simulink model "car_sim"  (R2023a)
settings: Solver=FixedStepAuto  StartTime=0.0  StopTime=20  FixedStep=.01  RelTol=1e-3
values from neighbouring files (symbols this model uses):
  cg = 13/12    (= 1.08333333333)    [car_script.m]    (also in car_script_FY_lookup.m; car_script_Pacejka4.m)
  chassis_k = 1000    [car_script.m]    (also in car_script_FY_lookup.m; car_script_Pacejka4.m)
  dist = zeros(1, length(road_height_right))    [car_script_FY_lookup.m]    (also in car_script_Pacejka4.m)
  f_anti = .2    (= 0.2)    [car_script.m]    (also in car_script_FY_lookup.m; car_script_Pacejka4.m)
  f_arb = 202.9*12    (= 2434.8)    [car_script.m]    (also in car_script_FY_lookup.m; car_script_Pacejka4.m)
  f_c = f_damp_ratio*(2*sqrt(f_sprung*f_spring/(32.17*2)))    [car_script.m]    (also in car_script_FY_lookup.m; car_script_Pacejka4.m)
  f_MR_arb = .4    (= 0.4)    [car_script.m]    (also in car_script_FY_lookup.m; car_script_Pacejka4.m)
  f_MR_spring = .99    (= 0.99)    [car_script.m]    (also in car_script_FY_lookup.m; car_script_Pacejka4.m)
  f_rc = 1/12    (= 0.0833333333333)    [car_script.m]    (also in car_script_FY_lookup.m; car_script_Pacejka4.m)
  f_spring = 250*12    (= 3000)    [car_script.m]    (also in car_script_FY_lookup.m; car_script_Pacejka4.m)
  f_sprung = total_weight*weight_distribution-f_unsprung    (= 276.76)    [car_script.m]    (also in car_script_FY_lookup.m; car_script_Pacejka4.m)
  f_unsprung = 48.24    [car_script.m]    (also in car_script_FY_lookup.m; car_script_Pacejka4.m)
  f_unsprung_cg = 6/12    (= 0.5)    [car_script.m]    (also in car_script_FY_lookup.m; car_script_Pacejka4.m)
  fy_slip_angle_lookup = [fy_slip_angle_lookup, -flip(fy_slip_angle_lookup(:,1:15),2)]    [car_script.m]    (also in car_script_FY_lookup.m)
  Izz = 500    [car_script.m]    (also in car_script_FY_lookup.m; car_script_Pacejka4.m)
  r_anti = .2    (= 0.2)    [car_script.m]    (also in car_script_FY_lookup.m; car_script_Pacejka4.m)
  r_arb = 108.66*12    (= 1303.92)    [car_script.m]    (also in car_script_FY_lookup.m; car_script_Pacejka4.m)
  r_c = r_damp_ratio*(2*sqrt(r_sprung*r_spring/(32.17*2)))    [car_script.m]    (also in car_script_FY_lookup.m; car_script_Pacejka4.m)
  r_MR_arb = .25    (= 0.25)    [car_script.m]    (also in car_script_FY_lookup.m; car_script_Pacejka4.m)
  r_MR_spring = .96    (= 0.96)    [car_script.m]    (also in car_script_FY_lookup.m; car_script_Pacejka4.m)
  r_rc = 2/12    (= 0.166666666667)    [car_script.m]    (also in car_script_FY_lookup.m; car_script_Pacejka4.m)
  r_spring = 150*12    (= 1800)    [car_script.m]    (also in car_script_FY_lookup.m; car_script_Pacejka4.m)
  r_sprung = total_weight*weight_distribution-r_unsprung    (= 277.44)    [car_script.m]    (also in car_script_FY_lookup.m; car_script_Pacejka4.m)
  r_unsprung = 47.56    [car_script.m]    (also in car_script_FY_lookup.m; car_script_Pacejka4.m)
  r_unsprung_cg = 6/12    (= 0.5)    [car_script.m]    (also in car_script_FY_lookup.m; car_script_Pacejka4.m)
  road_height_left = [zeros(1,10000)]    [car_script.m]    (also in car_script_FY_lookup.m; car_script_Pacejka4.m)
  road_height_right = [zeros(1,10000)]    [car_script.m]    (also in car_script_FY_lookup.m; car_script_Pacejka4.m)
  timestep = .01    (= 0.01)    [car_script.m]    (also in car_script_FY_lookup.m; car_script_Pacejka4.m)
  tire_c = .1*(2*sqrt(tire_k*f_unsprung/(2*32.17)))    [car_script.m]    (also in car_script_FY_lookup.m; car_script_Pacejka4.m)
  tire_k = 989*12    (= 11868)    [car_script.m]    (also in car_script_FY_lookup.m; car_script_Pacejka4.m)
  total_unsprung = f_unsprung + r_unsprung    (= 95.8)    [car_script.m]    (also in car_script_FY_lookup.m; car_script_Pacejka4.m)
  total_weight = 650    [car_script.m]    (also in car_script_FY_lookup.m; car_script_Pacejka4.m)
  track = 48/12    (= 4)    [car_script.m]    (also in car_script_FY_lookup.m; car_script_Pacejka4.m)
  vx_o = 51.3333    [car_script.m]    (also in car_script_FY_lookup.m; car_script_Pacejka4.m = 51.33)
  wheelbase = 60.5/12    (= 5.04166666667)    [car_script.m]    (also in car_script_FY_lookup.m; car_script_Pacejka4.m)
libraries: simulink_extras x1, simulink x1
(part 1 of 2)
settings Model: PauseTimes=1.01  Creator=truma  LastModifiedBy=truma
settings SolverCC: ZeroCrossAlgorithm=Adaptive
settings DebuggingCC: MaskedZcDiagnostic=none  IgnoredZcDiagnostic=none  ParameterPrecisionLossMsg=none  UnderSpecifiedDimensionMsg=warning

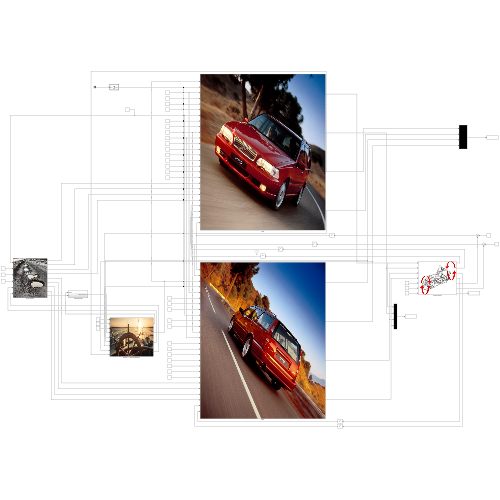
[thumbnail: Simulink's stored preview of the top-level diagram]
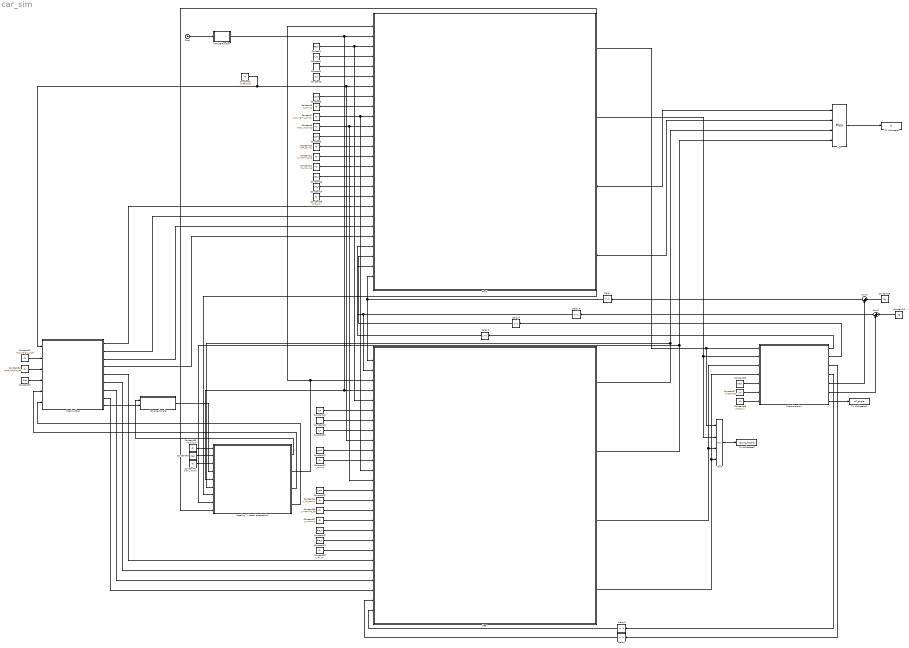
== system car_sim ==
  Chassis torsion : Subsystem
      mask Display: image('torsion.jpg'); % Use "Edit Image" on toolstrip to change.
  Clock : Clock
  Constant : Constant  Value=track
  Constant1 : Constant  Value=f_rc
  Constant10 : Constant  Value=f_MR_spring
  Constant11 : Constant  Value=f_unsprung_cg
  Constant12 : Constant  Value=f_unsprung
  Constant13 : Constant  Value=tire_k
  Constant14 : Constant  Value=tire_c
  Constant15 : Constant  Value=cg
  Constant16 : Constant  Value=f_MR_arb
  Constant18 : Constant  Value=r_rc
  Constant19 : Constant  Value=r_spring
  Constant2 : Constant  Value=f_spring
  Constant20 : Constant  Value=r_c
  Constant21 : Constant  Value=r_anti
  Constant22 : Constant  Value=r_sprung
  Constant23 : Constant  Value=cg
  Constant24 : Constant  Value=r_MR_spring
  Constant25 : Constant  Value=r_arb
  Constant26 : Constant  Value=r_unsprung_cg
  Constant27 : Constant  Value=r_unsprung
  Constant28 : Constant  Value=tire_k
  Constant29 : Constant  Value=tire_c
  Constant3 : Constant  Value=f_c
  Constant30 : Constant  Value=r_MR_arb
  Constant31 : Constant  Value=road_height_right
  Constant32 : Constant  Value=road_height_left
  Constant33 : Constant  Value=dist
  Constant36 : Constant  Value=track
  Constant37 : Constant  Value=wheelbase
  Constant38 : Constant  Value=chassis_k
  Constant39 : Constant  Value=wheelbase
  Constant4 : Constant  Value=wheelbase
  Constant40 : Constant  Value=track
  Constant41 : Constant  Value=total_weight
  Constant5 : Constant  Value=f_anti
  Constant6 : Constant  Value=f_sprung
  Constant7 : Constant  Value=f_sprung+r_sprung
  Constant8 : Constant  Value=total_unsprung
  Constant9 : Constant  Value=f_arb
  Delay : Delay  DelayLength=1  InitialCondition=cg
  Delay{2..5} (4 alike) : Delay  DelayLength=1
  Delay8 : Delay  DelayLength=1  InitialCondition=cg
  Front : Subsystem
      mask Display: image('front.jpg'); % Use "Edit Image" on toolstrip to change.
  MATLAB Function : MATLAB Function  TreatAsAtomicUnit=on
  Mux : Mux
  Mux1 : Mux
  Rear : Subsystem
      mask Display: image('rear.jpg'); % Use "Edit Image" on toolstrip to change.
  Road surface : Subsystem
      mask Display: image('pothole.jpg'); % Use "Edit Image" on toolstrip to change.
  Sum2 : Sum  Inputs=|++
  Sum3 : Sum  Inputs=|++
  To Workspace : ToWorkspace  VariableName=Fz  SaveFormat=Timeseries  SampleTime=-1
  To Workspace1 : ToWorkspace  VariableName=roll_angle  SaveFormat=Timeseries  SampleTime=-1
  To Workspace2 : ToWorkspace  VariableName=sprung_heights  SaveFormat=Timeseries  SampleTime=-1
  "steering -> lateral acceleration" : Subsystem
      mask Display: image('steering.jpeg'); % Use "Edit Image" on toolstrip to change.
  traversed angle : Subsystem
  wires:
  Front/2(sprung height FL) -> Mux1/2, Chassis torsion/2(sprung height FL)
  Rear/4(sprung height RL) -> Chassis torsion/4(sprung height RL), Mux1/4
  Chassis torsion/1(FR) -> Delay5/1
  Chassis torsion/2(FL) -> Delay4/1
  Chassis torsion/3(RR) -> Delay2/1
  Chassis torsion/4(RL) -> Delay3/1
  Constant/1 -> Rear/5(track), Front/3(track)
  Constant2/1 -> Front/5(front spring stiff)
  Constant3/1 -> Front/6(front damping coefficient)
  Constant5/1 -> Front/8(anti-squat)
  Constant6/1 -> Front/9(front sprung weight)
  Constant7/1 -> Front/10(total sprung weight), Rear/12(total sprung weight)
  Constant8/1 -> Front/11(total unsprung weight), Rear/13(total unsprung weight)
  Constant9/1 -> Front/12(front roll bar stiffness)
  Constant10/1 -> Front/13(front spring MR)
  Constant11/1 -> Front/14(front unsprung cg)
  Constant12/1 -> Front/15(front unsprung weight)
  Constant13/1 -> Front/16(front tire stiffness)
  Constant14/1 -> Front/17(front tire damping)
  Constant16/1 -> Front/18(front arb MR)
  Constant18/1 -> Rear/6(rear RC)
  Constant19/1 -> Rear/7(rear spring stiff)
  Constant20/1 -> Rear/8(rear damping coefficient)
  Constant21/1 -> Rear/10(anti-dive)
  Constant22/1 -> Rear/11(rear sprung weight)
  Constant25/1 -> Rear/14(rear roll bar stiffness)
  Constant24/1 -> Rear/15(rear spring MR)
  Constant26/1 -> Rear/16(rear unsprung cg)
  Constant27/1 -> Rear/17(rear unsprung weight)
  Constant28/1 -> Rear/18(rear tire stiffness)
  Constant29/1 -> Rear/19(rear tire damping)
  Constant30/1 -> Rear/20(rear arb MR)
  Road surface/1(FR_surface) -> Front/19(road height FR)
  Road surface/3(FL_surface) -> Front/21(road height FL)
  Road surface/7(RL_surface) -> Rear/23(road height RL)
  Road surface/5(RR_surface) -> Rear/21(road height RR)
  Road surface/2(FR_vel) -> Front/20(road velocity FR)
  Road surface/6(RR_vel) -> Rear/22(road velocity RR)
  Road surface/4(FL_vel) -> Front/22(road velocity FL)
  Road surface/8(RL_vel) -> Rear/24(road velocity RL)
  Constant31/1 -> Road surface/2(road height right)
  Constant32/1 -> Road surface/3(road height left)
  Constant33/1 -> Road surface/4(dist)
  Constant4/1 -> Road surface/1(wheelbase), Rear/9(wheelbase), Front/7(wheelbase)
  Front/4(Fz_FL) -> Mux/2, "steering -> lateral acceleration"/7(Fz_fl)
  Rear/1(Fz_RR) -> Mux/3, "steering -> lateral acceleration"/6(Fz_rr)
  Rear/2(Fz_RL) -> "steering -> lateral acceleration"/8(Fz_rl), Mux/4
  Mux/1 -> To Workspace/1
  Constant36/1 -> Chassis torsion/5(track)
  Constant38/1 -> Chassis torsion/7(chassis torsional stiffness)
  Constant37/1 -> Chassis torsion/6(wheelbase)
  Delay3/1 -> Rear/26(RL chassis force)
  Delay2/1 -> Rear/25(RR chassis force)
  Delay5/1 -> Front/23(FR chassis force)
  Delay4/1 -> Front/24(FL chassis force)
  Constant39/1 -> "steering -> lateral acceleration"/1(wheelbase)
  Constant40/1 -> "steering -> lateral acceleration"/2(track)
  Constant41/1 -> "steering -> lateral acceleration"/3(total_weight)
  Chassis torsion/7(roll) -> To Workspace1/1
  Clock/1 -> MATLAB Function/1(time)
  MATLAB Function/1(long_a) -> "steering -> lateral acceleration"/5(long_a), Rear/4(longitudinal a), Front/2(longitudinal a)
  Delay/1 -> Front/26(CG h), Rear/1(CG_front)
  Constant23/1 -> Sum2/1
  Sum2/1 -> Delay/1
  "steering -> lateral acceleration"/2(lat_a) -> Front/1(lateral a), Rear/3(lateral a)
  Chassis torsion/5(CG_f) -> Sum2/2
  Front/1(sprung height FR) -> Mux1/1, Chassis torsion/1(sprung height FR)
  Rear/3(sprung height RR) -> Mux1/3, Chassis torsion/3(sprung height RR)
  Mux1/1 -> To Workspace2/1
  Constant1/1 -> Front/4(front RC)
  Sum3/1 -> Delay8/1
  Constant15/1 -> Sum3/1
  Chassis torsion/6(CG_r) -> Sum3/2
  Delay8/1 -> Front/25(CG_rear), Rear/2(CG h)
  "steering -> lateral acceleration"/1(radius) -> traversed angle/1(radius)
  traversed angle/1(theta_world_frame) -> "steering -> lateral acceleration"/4(theta)
  Road surface/9(v) -> traversed angle/2(v)
  "steering -> lateral acceleration"/4(y_v) -> Road surface/6(y_v)
  "steering -> lateral acceleration"/3(x_v) -> Road surface/5(x_v)
  Front/3(Fz_FR) -> Mux/1, "steering -> lateral acceleration"/9(Fz_fr)

== system car_sim/Chassis torsion ==
  sprung height FR : Inport
  sprung height FL : Inport  Port=2
  sprung height RR : Inport  Port=3
  sprung height RL : Inport  Port=4
  track : Inport  Port=5
  wheelbase : Inport  Port=6
  chassis torsional stiffness : Inport  Port=7
  MATLAB Function : MATLAB Function  TreatAsAtomicUnit=on
  FR : Outport
  FL : Outport  Port=2
  RR : Outport  Port=3
  RL : Outport  Port=4
  CG_f : Outport  Port=5
  CG_r : Outport  Port=6
  roll : Outport  Port=7
  wires:
  sprung height FR/1 -> MATLAB Function/1(sprung_height_FR)
  sprung height FL/1 -> MATLAB Function/2(sprung_height_FL)
  sprung height RR/1 -> MATLAB Function/3(sprung_height_RR)
  sprung height RL/1 -> MATLAB Function/4(sprung_height_RL)
  track/1 -> MATLAB Function/5(track)
  wheelbase/1 -> MATLAB Function/7(wheelbase)
  chassis torsional stiffness/1 -> MATLAB Function/6(chassis_torsional_stiffness)
  MATLAB Function/2(FL) -> FL/1
  MATLAB Function/3(RR) -> RR/1
  MATLAB Function/4(RL) -> RL/1
  MATLAB Function/5(CG_f) -> CG_f/1
  MATLAB Function/7(roll) -> roll/1
  MATLAB Function/6(CG_r) -> CG_r/1
  MATLAB Function/1(FR) -> FR/1

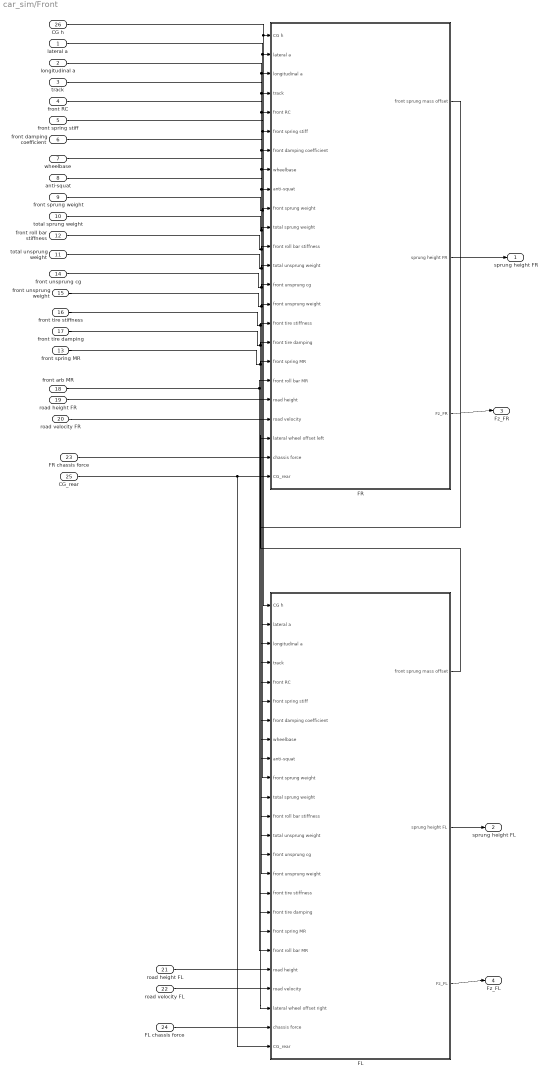
== system car_sim/Front ==
  lateral a : Inport
  longitudinal a : Inport  Port=2
  track : Inport  Port=3
  front RC : Inport  Port=4
  front spring stiff : Inport  Port=5
  front damping coefficient : Inport  Port=6
  wheelbase : Inport  Port=7
  anti-squat : Inport  Port=8
  front sprung weight : Inport  Port=9
  total sprung weight : Inport  Port=10
  total unsprung weight : Inport  Port=11
  front roll bar stiffness : Inport  Port=12
  front spring MR : Inport  Port=13
  front unsprung cg : Inport  Port=14
  front unsprung weight : Inport  Port=15
  front tire stiffness : Inport  Port=16
  front tire damping : Inport  Port=17
  front arb MR : Inport  Port=18
  road height FR : Inport  Port=19
  road velocity FR : Inport  Port=20
  road height FL : Inport  Port=21
  road velocity FL : Inport  Port=22
  FR chassis force : Inport  Port=23
  FL chassis force : Inport  Port=24
  CG_rear : Inport  Port=25
  CG h : Inport  Port=26
  FL : Subsystem
  FR : Subsystem
  sprung height FR : Outport
  sprung height FL : Outport  Port=2
  Fz_FR : Outport  Port=3
  Fz_FL : Outport  Port=4
  wires:
  CG h/1 -> FL/1(CG h), FR/1(CG h)
  lateral a/1 -> FL/2(lateral a), FR/2(lateral a)
  longitudinal a/1 -> FL/3(longitudinal a), FR/3(longitudinal a)
  track/1 -> FL/4(track), FR/4(track)
  front RC/1 -> FL/5(front RC), FR/5(front RC)
  front spring stiff/1 -> FL/6(front spring stiff), FR/6(front spring stiff)
  front damping coefficient/1 -> FL/7(front damping coefficient), FR/7(front damping coefficient)
  wheelbase/1 -> FL/8(wheelbase), FR/8(wheelbase)
  anti-squat/1 -> FL/9(anti-squat), FR/9(anti-squat)
  front sprung weight/1 -> FL/10(front sprung weight), FR/10(front sprung weight)
  total sprung weight/1 -> FL/11(total sprung weight), FR/11(total sprung weight)
  total unsprung weight/1 -> FL/13(total unsprung weight), FR/13(total unsprung weight)
  front roll bar stiffness/1 -> FL/12(front roll bar stiffness), FR/12(front roll bar stiffness)
  FR/1(front sprung mass offset) -> FL/22(lateral wheel offset right)
  front spring MR/1 -> FL/18(front spring MR), FR/18(front spring MR)
  front unsprung cg/1 -> FL/14(front unsprung cg), FR/14(front unsprung cg)
  front unsprung weight/1 -> FL/15(front unsprung weight), FR/15(front unsprung weight)
  front tire stiffness/1 -> FL/16(front tire stiffness), FR/16(front tire stiffness)
  front tire damping/1 -> FL/17(front tire damping), FR/17(front tire damping)
  front arb MR/1 -> FL/19(front roll bar MR), FR/19(front roll bar MR)
  FL/1(front sprung mass offset) -> FR/22(lateral wheel offset left)
  road height FR/1 -> FR/20(road height)
  road velocity FR/1 -> FR/21(road velocity)
  road height FL/1 -> FL/20(road height)
  road velocity FL/1 -> FL/21(road velocity)
  FR/2(sprung height FR) -> sprung height FR/1
  FL/2(sprung height FL) -> sprung height FL/1
  FR chassis force/1 -> FR/23(chassis force)
  FL chassis force/1 -> FL/23(chassis force)
  FR/3(Fz_FR) -> Fz_FR/1
  FL/3(Fz_FL) -> Fz_FL/1
  CG_rear/1 -> FL/24(CG_rear), FR/24(CG_rear)

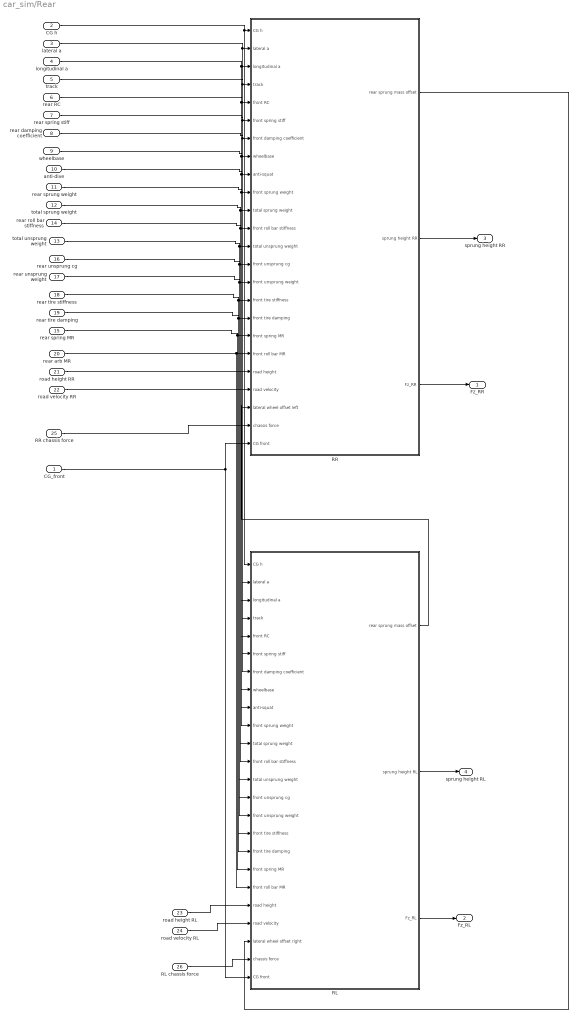
== system car_sim/Rear ==
  CG_front : Inport
  CG h : Inport  Port=2
  lateral a : Inport  Port=3
  longitudinal a : Inport  Port=4
  track : Inport  Port=5
  rear RC : Inport  Port=6
  rear spring stiff : Inport  Port=7
  rear damping coefficient : Inport  Port=8
  wheelbase : Inport  Port=9
  anti-dive : Inport  Port=10
  rear sprung weight : Inport  Port=11
  total sprung weight : Inport  Port=12
  total unsprung weight : Inport  Port=13
  rear roll bar stiffness : Inport  Port=14
  rear spring MR : Inport  Port=15
  rear unsprung cg : Inport  Port=16
  rear unsprung weight : Inport  Port=17
  rear tire stiffness : Inport  Port=18
  rear tire damping : Inport  Port=19
  rear arb MR : Inport  Port=20
  road height RR : Inport  Port=21
  road velocity RR : Inport  Port=22
  road height RL : Inport  Port=23
  road velocity RL : Inport  Port=24
  RR chassis force : Inport  Port=25
  RL chassis force : Inport  Port=26
  RL : Subsystem
  RR : Subsystem
  Fz_RR : Outport
  Fz_RL : Outport  Port=2
  sprung height RR : Outport  Port=3
  sprung height RL : Outport  Port=4
  wires:
  CG h/1 -> RL/1(CG h), RR/1(CG h)
  lateral a/1 -> RL/2(lateral a), RR/2(lateral a)
  longitudinal a/1 -> RL/3(longitudinal a), RR/3(longitudinal a)
  track/1 -> RL/4(track), RR/4(track)
  rear RC/1 -> RL/5(front RC), RR/5(front RC)
  rear spring stiff/1 -> RL/6(front spring stiff), RR/6(front spring stiff)
  rear damping coefficient/1 -> RL/7(front damping coefficient), RR/7(front damping coefficient)
  wheelbase/1 -> RL/8(wheelbase), RR/8(wheelbase)
  anti-dive/1 -> RL/9(anti-squat), RR/9(anti-squat)
  rear sprung weight/1 -> RL/10(front sprung weight), RR/10(front sprung weight)
  total sprung weight/1 -> RL/11(total sprung weight), RR/11(total sprung weight)
  total unsprung weight/1 -> RL/13(total unsprung weight), RR/13(total unsprung weight)
  rear roll bar stiffness/1 -> RL/12(front roll bar stiffness), RR/12(front roll bar stiffness)
  RR/1(rear sprung mass offset) -> RL/22(lateral wheel offset right)
  rear spring MR/1 -> RL/18(front spring MR), RR/18(front spring MR)
  rear unsprung cg/1 -> RL/14(front unsprung cg), RR/14(front unsprung cg)
  rear unsprung weight/1 -> RL/15(front unsprung weight), RR/15(front unsprung weight)
  rear tire stiffness/1 -> RL/16(front tire stiffness), RR/16(front tire stiffness)
  rear tire damping/1 -> RL/17(front tire damping), RR/17(front tire damping)
  rear arb MR/1 -> RL/19(front roll bar MR), RR/19(front roll bar MR)
  RL/1(rear sprung mass offset) -> RR/22(lateral wheel offset left)
  road height RR/1 -> RR/20(road height)
  road velocity RR/1 -> RR/21(road velocity)
  road height RL/1 -> RL/20(road height)
  road velocity RL/1 -> RL/21(road velocity)
  RR/2(sprung height RR) -> sprung height RR/1
  RL/2(sprung height RL) -> sprung height RL/1
  RR chassis force/1 -> RR/23(chassis force)
  RL chassis force/1 -> RL/23(chassis force)
  RR/3(Fz_RR) -> Fz_RR/1
  RL/3(Fz_RL) -> Fz_RL/1
  CG_front/1 -> RL/24(CG front), RR/24(CG front)

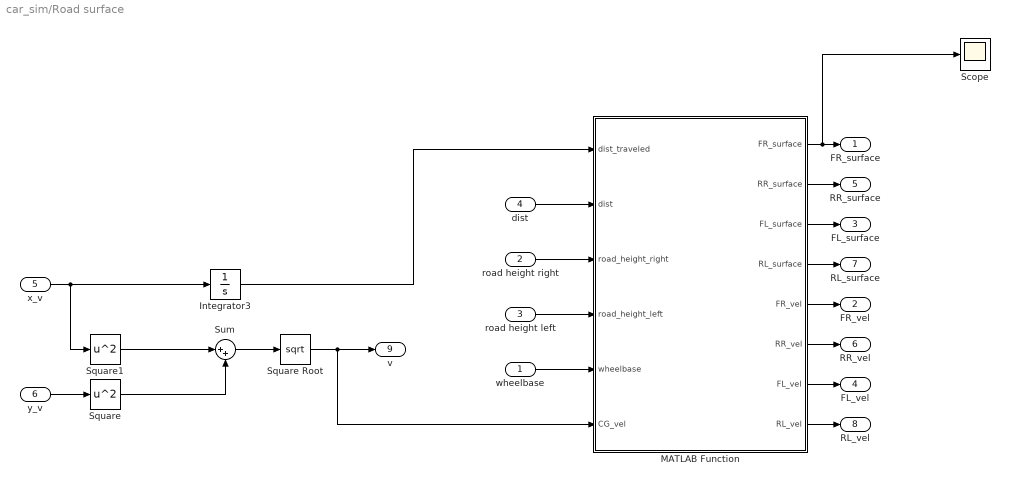
== system car_sim/Road surface ==
  wheelbase : Inport
  road height right : Inport  Port=2
  road height left : Inport  Port=3
  dist : Inport  Port=4
  x_v : Inport  Port=5
  y_v : Inport  Port=6
  Integrator3 : Integrator
  MATLAB Function : MATLAB Function  TreatAsAtomicUnit=on
  Scope : Scope
  Square : Math  Operator=square
  Square Root : Sqrt
  Square1 : Math  Operator=square
  Sum : Sum  Inputs=|++
  FR_surface : Outport
  FR_vel : Outport  Port=2
  FL_surface : Outport  Port=3
  FL_vel : Outport  Port=4
  RR_surface : Outport  Port=5
  RR_vel : Outport  Port=6
  RL_surface : Outport  Port=7
  RL_vel : Outport  Port=8
  v : Outport  Port=9
  wires:
  Integrator3/1 -> MATLAB Function/1(dist_traveled)
  road height right/1 -> MATLAB Function/3(road_height_right)
  road height left/1 -> MATLAB Function/4(road_height_left)
  dist/1 -> MATLAB Function/2(dist)
  wheelbase/1 -> MATLAB Function/5(wheelbase)
  MATLAB Function/1(FR_surface) -> FR_surface/1, Scope/1
  MATLAB Function/2(RR_surface) -> RR_surface/1
  MATLAB Function/3(FL_surface) -> FL_surface/1
  MATLAB Function/4(RL_surface) -> RL_surface/1
  x_v/1 -> Integrator3/1, Square1/1
  MATLAB Function/8(RL_vel) -> RL_vel/1
  MATLAB Function/7(FL_vel) -> FL_vel/1
  MATLAB Function/6(RR_vel) -> RR_vel/1
  MATLAB Function/5(FR_vel) -> FR_vel/1
  y_v/1 -> Square/1
  Square1/1 -> Sum/1
  Square/1 -> Sum/2
  Sum/1 -> Square Root/1
  Square Root/1 -> MATLAB Function/6(CG_vel), v/1

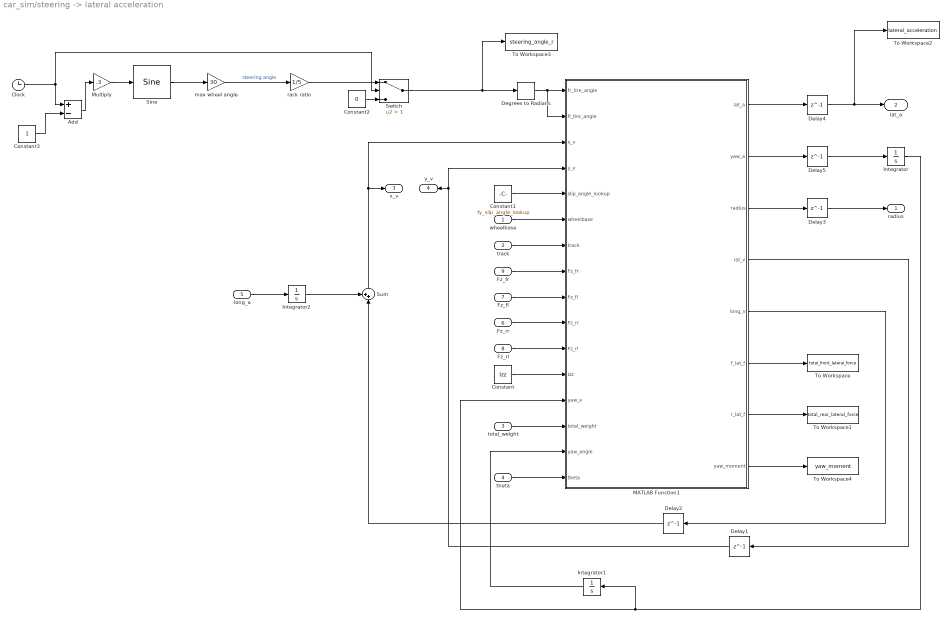
== system car_sim/steering -> lateral acceleration ==
  wheelbase : Inport
  track : Inport  Port=2
  total_weight : Inport  Port=3
  theta : Inport  Port=4
  long_a : Inport  Port=5
  Fz_rr : Inport  Port=6
  Fz_fl : Inport  Port=7
  Fz_rl : Inport  Port=8
  Fz_fr : Inport  Port=9
  Add : Sum  Inputs=+-
  Clock : Clock
  Constant : Constant  Value=Izz
  Constant1 : Constant  Value=fy_slip_angle_lookup
  Constant2 : Constant  Value=0
  Constant3 : Constant
  Degrees to Radians : simulink_extras/Transformations/Degrees to Radians
  Delay{1,3..5} (4 alike) : Delay  DelayLength=1
  Delay2 : Delay  DelayLength=1  InitialCondition=vx_o/2
  Integrator : Integrator
  Integrator1 : Integrator
  Integrator2 : Integrator
  MATLAB Function1 : MATLAB Function  TreatAsAtomicUnit=on
  Multiply : Gain  Gain=.3
  Sine : simulink/Lookup Tables/Sine  Formula=sin(2*pi*u)  NumDataPoints=(2^5)+1  OutputWordLength=16  InternalRulePriority=Speed
  Sum : Sum  Inputs=++|
  Switch : Switch  Criteria=u2 > Threshold  Threshold=1  SaturateOnIntegerOverflow=off  InputSameDT=off
  To Workspace : ToWorkspace  VariableName=total_front_lateral_force  SaveFormat=Timeseries  SampleTime=-1
  To Workspace1 : ToWorkspace  VariableName=total_rear_lateral_force  SaveFormat=Timeseries  SampleTime=-1
  To Workspace2 : ToWorkspace  VariableName=lateral_acceleration  SaveFormat=Timeseries  SampleTime=-1
  To Workspace3 : ToWorkspace  VariableName=steering_angle_r  SaveFormat=Timeseries  SampleTime=-1
  To Workspace4 : ToWorkspace  VariableName=yaw_moment  SaveFormat=Timeseries  SampleTime=-1
  max wheel angle : Gain  Gain=30
  rack ratio : Gain  Gain=1/5
  radius : Outport
  lat_a : Outport  Port=2
  x_v : Outport  Port=3
  y_v : Outport  Port=4
  wires:
  Multiply/1 -> Sine/1
  max wheel angle/1 -> rack ratio/1  "steering angle"
  Sine/1 -> max wheel angle/1
  Clock/1 -> Add/1, Switch/2
  Constant/1 -> MATLAB Function1/12(Izz)
  Constant1/1 -> MATLAB Function1/5(slip_angle_lookup)
  Fz_fr/1 -> MATLAB Function1/8(Fz_fr)
  wheelbase/1 -> MATLAB Function1/6(wheelbase)
  Fz_fl/1 -> MATLAB Function1/9(Fz_fl)
  MATLAB Function1/2(yaw_a) -> Delay5/1
  Integrator/1 -> MATLAB Function1/13(yaw_v), Integrator1/1
  total_weight/1 -> MATLAB Function1/14(total_weight)
  track/1 -> MATLAB Function1/7(track)
  rack ratio/1 -> Switch/1
  Constant2/1 -> Switch/3
  Constant3/1 -> Add/2
  Add/1 -> Multiply/1
  Switch/1 -> To Workspace3/1, Degrees to Radians/1
  MATLAB Function1/3(radius) -> Delay3/1
  MATLAB Function1/4(lat_v) -> Delay1/1
  Delay1/1 -> MATLAB Function1/4(y_v), y_v/1
  MATLAB Function1/5(long_v) -> Delay2/1
  long_a/1 -> Integrator2/1
  Delay2/1 -> Sum/2
  Integrator2/1 -> Sum/1
  Sum/1 -> x_v/1, MATLAB Function1/3(x_v)
  Delay3/1 -> radius/1
  Delay4/1 -> To Workspace2/1, lat_a/1
  MATLAB Function1/1(lat_a) -> Delay4/1
  Delay5/1 -> Integrator/1
  theta/1 -> MATLAB Function1/16(theta)
  MATLAB Function1/6(f_lat_f) -> To Workspace/1
  MATLAB Function1/7(r_lat_f) -> To Workspace1/1
  Fz_rr/1 -> MATLAB Function1/10(Fz_rr)
  Fz_rl/1 -> MATLAB Function1/11(Fz_rl)
  Integrator1/1 -> MATLAB Function1/15(yaw_angle)
  Degrees to Radians/1 -> MATLAB Function1/2(fl_tire_angle), MATLAB Function1/1(fr_tire_angle)
  MATLAB Function1/8(yaw_moment) -> To Workspace4/1

== system car_sim/traversed angle ==
  radius : Inport
  v : Inport  Port=2
  Delay : Delay  DelayLength=1
  Divide : Product  Inputs=*/
  Gain : Gain  Gain=timestep
  MATLAB Function : MATLAB Function  TreatAsAtomicUnit=on
  Sum : Sum  Inputs=|++
  theta_world_frame : Outport
  wires:
  v/1 -> Gain/1
  Gain/1 -> Divide/1
  Delay/1 -> Sum/2
  Divide/1 -> Sum/1
  MATLAB Function/1(y) -> Divide/2
  Sum/1 -> Delay/1, theta_world_frame/1
  radius/1 -> MATLAB Function/1(u)

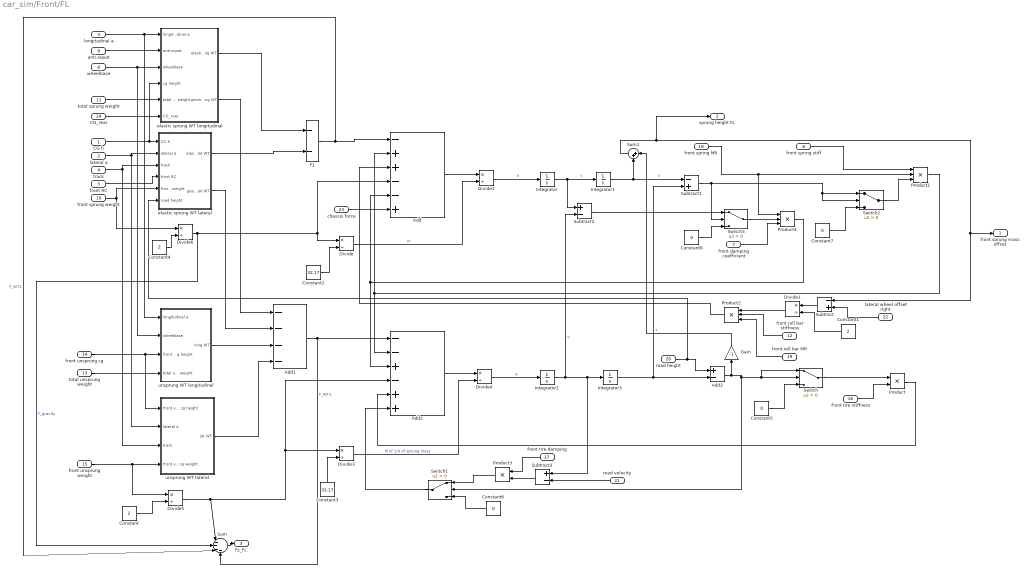
== system car_sim/Front/FL ==
  CG h : Inport
  lateral a : Inport  Port=2
  longitudinal a : Inport  Port=3
  track : Inport  Port=4
  front RC : Inport  Port=5
  front spring stiff : Inport  Port=6
  front damping coefficient : Inport  Port=7
  wheelbase : Inport  Port=8
  anti-squat : Inport  Port=9
  front sprung weight : Inport  Port=10
  total sprung weight : Inport  Port=11
  front roll bar stiffness : Inport  Port=12
  total unsprung weight : Inport  Port=13
  front unsprung cg : Inport  Port=14
  front unsprung weight : Inport  Port=15
  front tire stiffness : Inport  Port=16
  front tire damping : Inport  Port=17
  front spring MR : Inport  Port=18
  front roll bar MR : Inport  Port=19
  road height : Inport  Port=20
  road velocity : Inport  Port=21
  lateral wheel offset right : Inport  Port=22
  chassis force : Inport  Port=23
  CG_rear : Inport  Port=24
  " unsprung WT longitudinal" : Subsystem
  Add : Sum  Inputs=-++--+
  Add1 : Sum  Inputs=----
  Add2 : Sum  Inputs=--+-++
  Add3 : Sum  Inputs=+-
  Constant : Constant  Value=2
  Constant1 : Constant  Value=2
  Constant2 : Constant  Value=32.17
  Constant3 : Constant  Value=32.17
  Constant4 : Constant  Value=2
  Constant{5..8} (4 alike) : Constant  Value=0
  Divide{,1..6} (7 alike) : Product  Inputs=*/
  F1 : Sum  Inputs=--
  Gain : Gain  Gain=-1
  Integrator{,1..3} (4 alike) : Integrator
  Product : Product
  Product1 : Product  Inputs=3
  Product2 : Product  Inputs=3
  Product3 : Product
  Product4 : Product  Inputs=3
  Subtract : Sum  Inputs=-+
  Subtract1 : Sum  Inputs=-+
  Subtract2 : Sum  Inputs=+-
  Subtract3 : Sum  Inputs=+-
  Sum : Sum  Inputs=|----
  Sum1 : Sum  Inputs=|++
  Switch{,1..3} (4 alike) : Switch  Criteria=u2 > Threshold  SaturateOnIntegerOverflow=off  InputSameDT=off
  elastic sprung WT lateral : Subsystem
  elastic sprung WT longitudinal : Subsystem
  unsprung WT lateral : Subsystem
  front sprung mass offset : Outport
  sprung height FL : Outport  Port=2
  Fz_FL : Outport  Port=3
  wires:
  CG h/1 -> elastic sprung WT longitudinal/4(cg height), elastic sprung WT lateral/1(CG h)
  F1/1 -> Sum/3, Add/1  "F_WT2"
  lateral a/1 -> unsprung WT lateral/2(lateral a), elastic sprung WT lateral/2(lateral a)
  elastic sprung WT longitudinal/1(elastic long WT) -> F1/1
  wheelbase/1 -> " unsprung WT longitudinal"/2(wheelbase), elastic sprung WT longitudinal/3(wheelbase)
  anti-squat/1 -> elastic sprung WT longitudinal/2(anti-squat)
  longitudinal a/1 -> " unsprung WT longitudinal"/1(longitudinal a), elastic sprung WT longitudinal/1(longitudinal a)
  front damping coefficient/1 -> Product4/3
  lateral wheel offset right/1 -> Subtract/2
  front RC/1 -> elastic sprung WT lateral/4(front RC)
  track/1 -> unsprung WT lateral/3(track), elastic sprung WT lateral/3(track)
  front roll bar stiffness/1 -> Product2/2
  elastic sprung WT lateral/1(elastic lat WT) -> F1/2
  front spring stiff/1 -> Product1/1
  Subtract/1 -> Divide1/1
  Constant1/1 -> Divide1/2
  Divide1/1 -> Product2/1
  front sprung weight/1 -> Divide6/1, elastic sprung WT lateral/5(front sprung weight)
  Constant2/1 -> Divide/2
  Divide/1 -> Divide2/2  "m"
  Add/1 -> Divide2/1
  Divide2/1 -> Integrator/1  "a"
  Integrator/1 -> Subtract2/1, Integrator1/1  "v"
  Integrator1/1 -> Subtract1/1, Sum1/2  "x"
  total unsprung weight/1 -> " unsprung WT longitudinal"/4(total unsprung weight)
  front unsprung cg/1 -> unsprung WT lateral/1(front unsprung cg height), " unsprung WT longitudinal"/3(front unsprung weight cg height)
  elastic sprung WT longitudinal/2(geom long WT) -> Add1/1
  elastic sprung WT lateral/2(geom lat WT) -> Add1/2
  " unsprung WT longitudinal"/1(long WT) -> Add1/3
  unsprung WT lateral/1(lat WT) -> Add1/4
  Add1/1 -> Sum/4, Add2/1  "F_WT1"
  Constant3/1 -> Divide3/2
  Divide3/1 -> Divide4/2  "M of 1/4 of sprung mass"
  Add2/1 -> Divide4/1
  front unsprung weight/1 -> Divide5/1, unsprung WT lateral/4(front unsprung weight)
  Constant/1 -> Divide5/2
  Divide5/1 -> Add2/4, Divide3/1, Sum/1
  Constant4/1 -> Divide6/2
  Divide6/1 -> Sum/2, Add/4, Divide/1  "F_gravity"
  Divide4/1 -> Integrator2/1  "a"
  Integrator2/1 -> Subtract2/2, Subtract3/1, Integrator3/1  "v"
  Integrator3/1 -> Subtract1/2, Add3/2  "x"
  front spring MR/1 -> Product4/1, Product1/2
  front roll bar MR/1 -> Product2/3
  Product2/1 -> Add/3
  Product4/1 -> Add2/3, Add/5
  Product1/1 -> Add2/2, Add/2
  road height/1 -> elastic sprung WT lateral/6(road height), Add3/1
  front tire stiffness/1 -> Product/2
  Product/1 -> Add2/5
  road velocity/1 -> Subtract3/2
  Subtract3/1 -> Product3/2
  front tire damping/1 -> Product3/1
  Constant5/1 -> Switch/3
  Switch/1 -> Product/1
  Constant6/1 -> Switch1/3
  Add3/1 -> Switch1/2, Switch/1, Switch/2, Gain/1
  Product3/1 -> Switch1/1
  Switch1/1 -> Add2/6
  Subtract1/1 -> Switch2/2, Switch2/1, Switch3/2
  Constant7/1 -> Switch2/3
  Switch2/1 -> Product1/3
  Constant8/1 -> Switch3/3
  Subtract2/1 -> Switch3/1
  Switch3/1 -> Product4/2
  Sum/1 -> Fz_FL/1
  Sum1/1 -> front sprung mass offset/1, Subtract/1, sprung height FL/1
  chassis force/1 -> Add/6
  CG_rear/1 -> elastic sprung WT longitudinal/6(CG_rear)
  total sprung weight/1 -> elastic sprung WT longitudinal/5(total sprung weight)
  Gain/1 -> Sum1/1

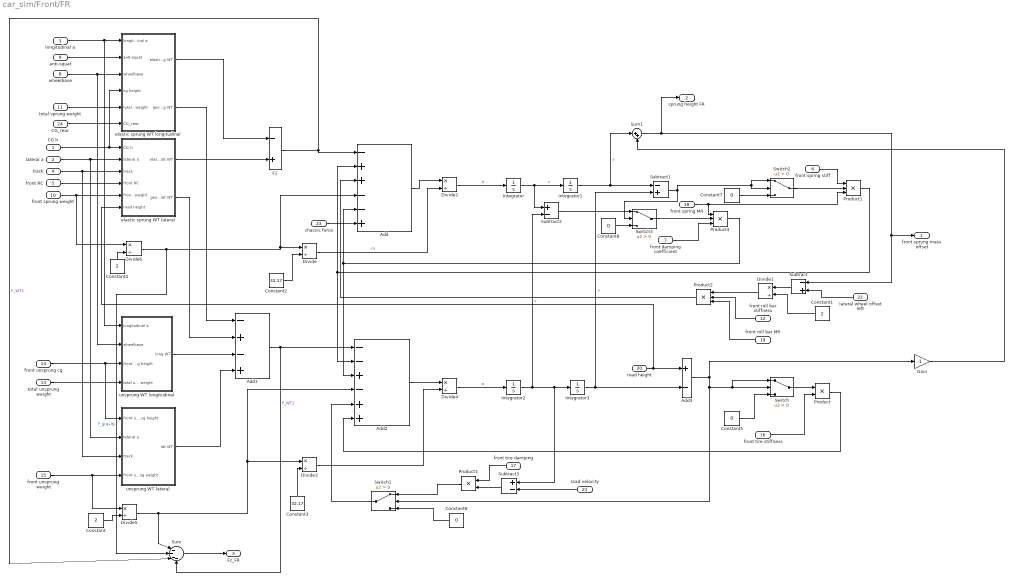
== system car_sim/Front/FR ==
  CG h : Inport
  lateral a : Inport  Port=2
  longitudinal a : Inport  Port=3
  track : Inport  Port=4
  front RC : Inport  Port=5
  front spring stiff : Inport  Port=6
  front damping coefficient : Inport  Port=7
  wheelbase : Inport  Port=8
  anti-squat : Inport  Port=9
  front sprung weight : Inport  Port=10
  total sprung weight : Inport  Port=11
  front roll bar stiffness : Inport  Port=12
  total unsprung weight : Inport  Port=13
  front unsprung cg : Inport  Port=14
  front unsprung weight : Inport  Port=15
  front tire stiffness : Inport  Port=16
  front tire damping : Inport  Port=17
  front spring MR : Inport  Port=18
  front roll bar MR : Inport  Port=19
  road height : Inport  Port=20
  road velocity : Inport  Port=21
  lateral wheel offset left : Inport  Port=22
  chassis force : Inport  Port=23
  CG_rear : Inport  Port=24
  " unsprung WT longitudinal" : Subsystem
  Add : Sum  Inputs=-++--+
  Add1 : Sum  Inputs=-+-+
  Add2 : Sum  Inputs=--+-++
  Add3 : Sum  Inputs=+-
  Constant : Constant  Value=2
  Constant1 : Constant  Value=2
  Constant2 : Constant  Value=32.17
  Constant3 : Constant  Value=32.17
  Constant4 : Constant  Value=2
  Constant{5..8} (4 alike) : Constant  Value=0
  Divide{,1..6} (7 alike) : Product  Inputs=*/
  F1 : Sum  Inputs=-+
  Gain : Gain  Gain=-1
  Integrator{,1..3} (4 alike) : Integrator
  Product : Product
  Product1 : Product  Inputs=3
  Product2 : Product  Inputs=3
  Product3 : Product
  Product4 : Product  Inputs=3
  Subtract : Sum  Inputs=-+
  Subtract1 : Sum  Inputs=-+
  Subtract2 : Sum  Inputs=+-
  Subtract3 : Sum  Inputs=+-
  Sum : Sum  Inputs=|----
  Sum1 : Sum  Inputs=|++
  Switch{,1..3} (4 alike) : Switch  Criteria=u2 > Threshold  SaturateOnIntegerOverflow=off  InputSameDT=off
  elastic sprung WT lateral : Subsystem
  elastic sprung WT longitudinal : Subsystem
  unsprung WT lateral : Subsystem
  front sprung mass offset : Outport
  sprung height FR : Outport  Port=2
  Fz_FR : Outport  Port=3
  wires:
  CG h/1 -> elastic sprung WT longitudinal/4(cg height), elastic sprung WT lateral/1(CG h)
  F1/1 -> Sum/3, Add/1  "F_WT2"
  lateral a/1 -> unsprung WT lateral/2(lateral a), elastic sprung WT lateral/2(lateral a)
  elastic sprung WT longitudinal/1(elastic long WT) -> F1/1
  wheelbase/1 -> " unsprung WT longitudinal"/2(wheelbase), elastic sprung WT longitudinal/3(wheelbase)
  anti-squat/1 -> elastic sprung WT longitudinal/2(anti-squat)
  longitudinal a/1 -> " unsprung WT longitudinal"/1(longitudinal a), elastic sprung WT longitudinal/1(longitudinal a)
  front damping coefficient/1 -> Product4/3
  lateral wheel offset left/1 -> Subtract/2
  front RC/1 -> elastic sprung WT lateral/4(front RC)
  track/1 -> unsprung WT lateral/3(track), elastic sprung WT lateral/3(track)
  front roll bar stiffness/1 -> Product2/2
  front spring stiff/1 -> Product1/1
  Subtract/1 -> Divide1/1
  Constant1/1 -> Divide1/2
  Divide1/1 -> Product2/1
  front sprung weight/1 -> Divide6/1, elastic sprung WT lateral/5(front sprung weight)
  Constant2/1 -> Divide/2
  Divide/1 -> Divide2/2  "m"
  Add/1 -> Divide2/1
  Divide2/1 -> Integrator/1  "a"
  Integrator/1 -> Subtract2/1, Integrator1/1  "v"
  Integrator1/1 -> Sum1/1, Subtract1/1  "x"
  total unsprung weight/1 -> " unsprung WT longitudinal"/4(total unsprung weight)
  front unsprung cg/1 -> unsprung WT lateral/1(front unsprung cg height), " unsprung WT longitudinal"/3(front unsprung weight cg height)
  elastic sprung WT longitudinal/2(geom long WT) -> Add1/1
  elastic sprung WT lateral/2(geom lat WT) -> Add1/2
  " unsprung WT longitudinal"/1(long WT) -> Add1/3
  unsprung WT lateral/1(lat WT) -> Add1/4
  Add1/1 -> Add2/1, Sum/4  "F_WT1"
  Constant3/1 -> Divide3/2
  Divide3/1 -> Divide4/2
  Add2/1 -> Divide4/1
  front unsprung weight/1 -> Divide5/1, unsprung WT lateral/4(front unsprung weight)
  Constant/1 -> Divide5/2
  Divide5/1 -> Add2/4, Divide3/1, Sum/1
  Constant4/1 -> Divide6/2
  Divide6/1 -> Sum/2, Add/4, Divide/1  "F_gravity"
  Divide4/1 -> Integrator2/1  "a"
  Integrator2/1 -> Subtract2/2, Subtract3/1, Integrator3/1  "v"
  Integrator3/1 -> Add3/2, Subtract1/2  "x"
  front roll bar MR/1 -> Product2/3
  Product2/1 -> Add/3
  Product4/1 -> Add2/3, Add/5
  Product1/1 -> Add2/2, Add/2
  road height/1 -> elastic sprung WT lateral/6(road height), Add3/1
  front tire stiffness/1 -> Product/2
  Product/1 -> Add2/6
  road velocity/1 -> Subtract3/2
  Subtract3/1 -> Product3/2
  front tire damping/1 -> Product3/1
  Constant5/1 -> Switch/3
  Switch/1 -> Product/1
  Add3/1 -> Gain/1, Switch1/2, Switch/1, Switch/2
  Constant6/1 -> Switch1/3
  Product3/1 -> Switch1/1
  Switch1/1 -> Add2/5
  Constant7/1 -> Switch2/3
  Switch2/1 -> Product1/2
  Constant8/1 -> Switch3/3
  Subtract1/1 -> Switch2/2, Switch2/1, Switch3/2
  Switch3/1 -> Product4/2
  Subtract2/1 -> Switch3/1
  front spring MR/1 -> Product4/1, Product1/3
  Sum/1 -> Fz_FR/1
  Sum1/1 -> Subtract/1, front sprung mass offset/1, sprung height FR/1
  elastic sprung WT lateral/1(elastic lat WT) -> F1/2
  chassis force/1 -> Add/6
  CG_rear/1 -> elastic sprung WT longitudinal/6(CG_rear)
  total sprung weight/1 -> elastic sprung WT longitudinal/5(total sprung weight)
  Gain/1 -> Sum1/2

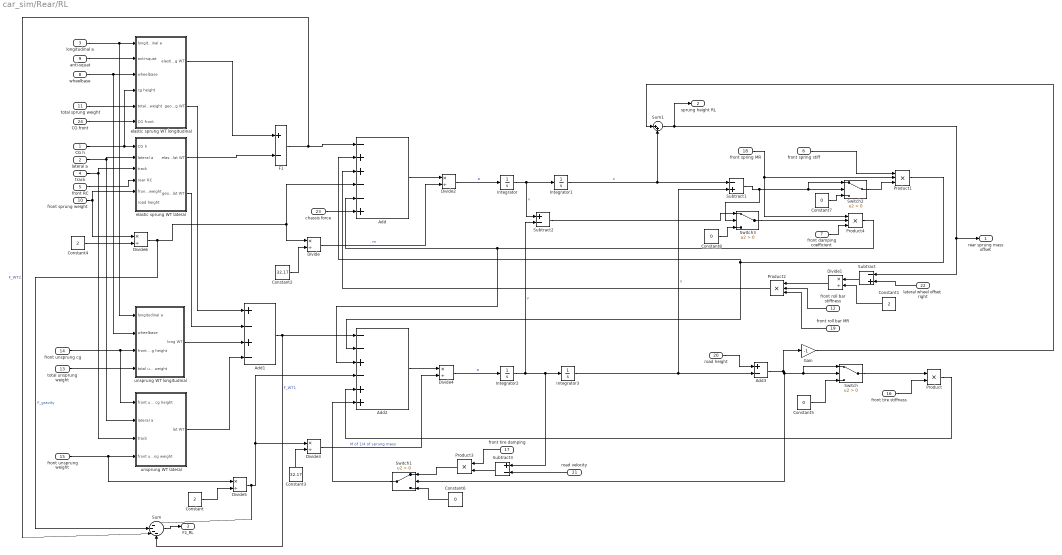
== system car_sim/Rear/RL ==
  CG h : Inport
  lateral a : Inport  Port=2
  longitudinal a : Inport  Port=3
  track : Inport  Port=4
  front RC : Inport  Port=5
  front spring stiff : Inport  Port=6
  front damping coefficient : Inport  Port=7
  wheelbase : Inport  Port=8
  anti-squat : Inport  Port=9
  front sprung weight : Inport  Port=10
  total sprung weight : Inport  Port=11
  front roll bar stiffness : Inport  Port=12
  total unsprung weight : Inport  Port=13
  front unsprung cg : Inport  Port=14
  front unsprung weight : Inport  Port=15
  front tire stiffness : Inport  Port=16
  front tire damping : Inport  Port=17
  front spring MR : Inport  Port=18
  front roll bar MR : Inport  Port=19
  road height : Inport  Port=20
  road velocity : Inport  Port=21
  lateral wheel offset right : Inport  Port=22
  chassis force : Inport  Port=23
  CG front : Inport  Port=24
  " unsprung WT longitudinal" : Subsystem
  Add : Sum  Inputs=-++--+
  Add1 : Sum  Inputs=+-+-
  Add2 : Sum  Inputs=--+-++
  Add3 : Sum  Inputs=+-
  Constant : Constant  Value=2
  Constant1 : Constant  Value=2
  Constant2 : Constant  Value=32.17
  Constant3 : Constant  Value=32.17
  Constant4 : Constant  Value=2
  Constant{5..8} (4 alike) : Constant  Value=0
  Divide{,1..6} (7 alike) : Product  Inputs=*/
  F1 : Sum  Inputs=+-
  Gain : Gain  Gain=-1
  Integrator{,1..3} (4 alike) : Integrator
  Product : Product
  Product1 : Product  Inputs=3
  Product2 : Product  Inputs=3
  Product3 : Product
  Product4 : Product  Inputs=3
  Subtract : Sum  Inputs=-+
  Subtract1 : Sum  Inputs=-+
  Subtract2 : Sum  Inputs=+-
  Subtract3 : Sum  Inputs=+-
  Sum : Sum  Inputs=|----
  Sum1 : Sum  Inputs=|++
  Switch{,1..3} (4 alike) : Switch  Criteria=u2 > Threshold  SaturateOnIntegerOverflow=off  InputSameDT=off
  elastic sprung WT lateral : Subsystem
  elastic sprung WT longitudinal : Subsystem
  unsprung WT lateral : Subsystem
  rear sprung mass offset : Outport
  sprung height RL : Outport  Port=2
  Fz_RL : Outport  Port=3
  wires:
  CG h/1 -> elastic sprung WT longitudinal/4(cg height), elastic sprung WT lateral/1(CG h)
  F1/1 -> Sum/3, Add/1  "F_WT2"
  lateral a/1 -> unsprung WT lateral/2(lateral a), elastic sprung WT lateral/2(lateral a)
  elastic sprung WT longitudinal/1(elastic long WT) -> F1/1
  wheelbase/1 -> " unsprung WT longitudinal"/2(wheelbase), elastic sprung WT longitudinal/3(wheelbase)
  anti-squat/1 -> elastic sprung WT longitudinal/2(anti-squat)
  longitudinal a/1 -> " unsprung WT longitudinal"/1(longitudinal a), elastic sprung WT longitudinal/1(longitudinal a)
  front damping coefficient/1 -> Product4/3
  lateral wheel offset right/1 -> Subtract/2
  front RC/1 -> elastic sprung WT lateral/4(rear RC)
  track/1 -> unsprung WT lateral/3(track), elastic sprung WT lateral/3(track)
  front roll bar stiffness/1 -> Product2/2
  total sprung weight/1 -> elastic sprung WT longitudinal/5(total sprung weight)
  elastic sprung WT lateral/1(elastic lat WT) -> F1/2
  front spring stiff/1 -> Product1/1
  Subtract/1 -> Divide1/1
  Constant1/1 -> Divide1/2
  Divide1/1 -> Product2/1
  front sprung weight/1 -> Divide6/1, elastic sprung WT lateral/5(front sprung weight)
  Constant2/1 -> Divide/2
  Divide/1 -> Divide2/2  "m"
  Add/1 -> Divide2/1
  Divide2/1 -> Integrator/1  "a"
  Integrator/1 -> Subtract2/1, Integrator1/1  "v"
  Integrator1/1 -> Subtract1/1, Sum1/2  "x"
  total unsprung weight/1 -> " unsprung WT longitudinal"/4(total unsprung weight)
  front unsprung cg/1 -> unsprung WT lateral/1(front unsprung cg height), " unsprung WT longitudinal"/3(front unsprung weight cg height)
  elastic sprung WT longitudinal/2(geom long WT) -> Add1/1
  elastic sprung WT lateral/2(geom lat WT) -> Add1/2
  " unsprung WT longitudinal"/1(long WT) -> Add1/3
  unsprung WT lateral/1(lat WT) -> Add1/4
  Add1/1 -> Sum/4, Add2/1  "F_WT1"
  Constant3/1 -> Divide3/2
  Divide3/1 -> Divide4/2  "M of 1/4 of sprung mass"
  Add2/1 -> Divide4/1
  front unsprung weight/1 -> Divide5/1, unsprung WT lateral/4(front unsprung weight)
  Constant/1 -> Divide5/2
  Constant4/1 -> Divide6/2
  Divide6/1 -> Sum/2, Add/4, Divide/1  "F_gravity"
  Divide4/1 -> Integrator2/1  "a"
  Integrator2/1 -> Subtract2/2, Subtract3/1, Integrator3/1  "v"
  Integrator3/1 -> Subtract1/2, Add3/2  "x"
  front spring MR/1 -> Product1/2, Product4/1
  front roll bar MR/1 -> Product2/3
  Product2/1 -> Add/3
  Product4/1 -> Add2/3, Add/5
  Product1/1 -> Add2/2, Add/2
  road height/1 -> Add3/1
  front tire stiffness/1 -> Product/2
  Product/1 -> Add2/5
  road velocity/1 -> Subtract3/2
  Subtract3/1 -> Product3/2
  front tire damping/1 -> Product3/1
  Constant5/1 -> Switch/3
  Switch/1 -> Product/1
  Constant6/1 -> Switch1/3
  Add3/1 -> Gain/1, Switch1/2, Switch/1, Switch/2
  Product3/1 -> Switch1/1
  Switch1/1 -> Add2/6
  Constant7/1 -> Switch2/3
  Switch2/1 -> Product1/3
  Constant8/1 -> Switch3/3
  Switch3/1 -> Product4/2
  Sum/1 -> Fz_RL/1
  Divide5/1 -> Sum/1, Add2/4, Divide3/1
  Sum1/1 -> rear sprung mass offset/1, Subtract/1, sprung height RL/1
  Subtract1/1 -> Switch3/2, Switch2/1, Switch2/2
  Subtract2/1 -> Switch3/1
  chassis force/1 -> Add/6
  CG front/1 -> elastic sprung WT longitudinal/6(CG front)
  Gain/1 -> Sum1/1

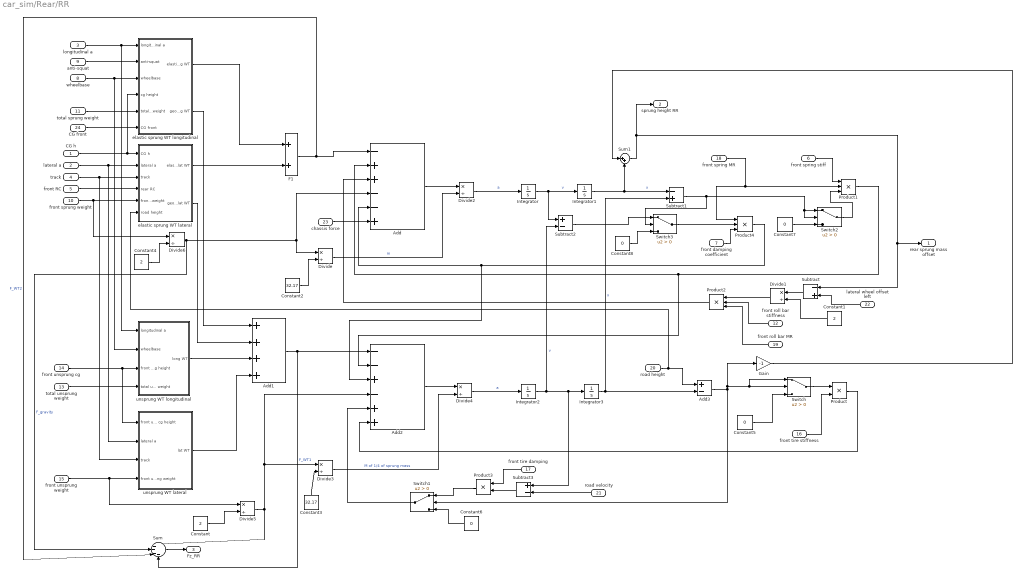
== system car_sim/Rear/RR ==
  CG h : Inport
  lateral a : Inport  Port=2
  longitudinal a : Inport  Port=3
  track : Inport  Port=4
  front RC : Inport  Port=5
  front spring stiff : Inport  Port=6
  front damping coefficient : Inport  Port=7
  wheelbase : Inport  Port=8
  anti-squat : Inport  Port=9
  front sprung weight : Inport  Port=10
  total sprung weight : Inport  Port=11
  front roll bar stiffness : Inport  Port=12
  total unsprung weight : Inport  Port=13
  front unsprung cg : Inport  Port=14
  front unsprung weight : Inport  Port=15
  front tire stiffness : Inport  Port=16
  front tire damping : Inport  Port=17
  front spring MR : Inport  Port=18
  front roll bar MR : Inport  Port=19
  road height : Inport  Port=20
  road velocity : Inport  Port=21
  lateral wheel offset left : Inport  Port=22
  chassis force : Inport  Port=23
  CG front : Inport  Port=24
  " unsprung WT longitudinal" : Subsystem
  Add : Sum  Inputs=-++--+
  Add1 : Sum  Inputs=++++
  Add2 : Sum  Inputs=--+-++
  Add3 : Sum  Inputs=+-
  Constant : Constant  Value=2
  Constant1 : Constant  Value=2
  Constant2 : Constant  Value=32.17
  Constant3 : Constant  Value=32.17
  Constant4 : Constant  Value=2
  Constant{5..8} (4 alike) : Constant  Value=0
  Divide{,1..6} (7 alike) : Product  Inputs=*/
  F1 : Sum
  Gain : Gain  Gain=-1
  Integrator{,1..3} (4 alike) : Integrator
  Product : Product
  Product1 : Product  Inputs=3
  Product2 : Product  Inputs=3
  Product3 : Product
  Product4 : Product  Inputs=3
  Subtract : Sum  Inputs=-+
  Subtract1 : Sum  Inputs=-+
  Subtract2 : Sum  Inputs=+-
  Subtract3 : Sum  Inputs=+-
  Sum : Sum  Inputs=|----
  Sum1 : Sum  Inputs=|++
  Switch{,1..3} (4 alike) : Switch  Criteria=u2 > Threshold  SaturateOnIntegerOverflow=off  InputSameDT=off
  elastic sprung WT lateral : Subsystem
  elastic sprung WT longitudinal : Subsystem
  unsprung WT lateral : Subsystem
  rear sprung mass offset : Outport
  sprung height RR : Outport  Port=2
  Fz_RR : Outport  Port=3
  wires:
  CG h/1 -> elastic sprung WT longitudinal/4(cg height), elastic sprung WT lateral/1(CG h)
  F1/1 -> Sum/3, Add/1  "F_WT2"
  lateral a/1 -> unsprung WT lateral/2(lateral a), elastic sprung WT lateral/2(lateral a)
  elastic sprung WT longitudinal/1(elastic long WT) -> F1/1
  wheelbase/1 -> " unsprung WT longitudinal"/2(wheelbase), elastic sprung WT longitudinal/3(wheelbase)
  anti-squat/1 -> elastic sprung WT longitudinal/2(anti-squat)
  longitudinal a/1 -> " unsprung WT longitudinal"/1(longitudinal a), elastic sprung WT longitudinal/1(longitudinal a)
  front damping coefficient/1 -> Product4/3
  lateral wheel offset left/1 -> Subtract/2
  front RC/1 -> elastic sprung WT lateral/4(rear RC)
  track/1 -> unsprung WT lateral/3(track), elastic sprung WT lateral/3(track)
  front roll bar stiffness/1 -> Product2/2
  total sprung weight/1 -> elastic sprung WT longitudinal/5(total sprung weight)
  front spring stiff/1 -> Product1/1
  Subtract/1 -> Divide1/1
  Constant1/1 -> Divide1/2
  Divide1/1 -> Product2/1
  front sprung weight/1 -> Divide6/1, elastic sprung WT lateral/5(front sprung weight)
  Constant2/1 -> Divide/2
  Divide/1 -> Divide2/2  "m"
  Divide2/1 -> Integrator/1  "a"
  Integrator/1 -> Subtract2/1, Integrator1/1  "v"
  Integrator1/1 -> Sum1/2, Subtract1/1  "x"
  total unsprung weight/1 -> " unsprung WT longitudinal"/4(total unsprung weight)
  front unsprung cg/1 -> unsprung WT lateral/1(front unsprung cg height), " unsprung WT longitudinal"/3(front unsprung weight cg height)
  elastic sprung WT longitudinal/2(geom long WT) -> Add1/1
  elastic sprung WT lateral/2(geom lat WT) -> Add1/2
  " unsprung WT longitudinal"/1(long WT) -> Add1/3
  unsprung WT lateral/1(lat WT) -> Add1/4
  Add1/1 -> Sum/4, Add2/1  "F_WT1"
  Constant3/1 -> Divide3/2
  Divide3/1 -> Divide4/2  "M of 1/4 of sprung mass"
  Add2/1 -> Divide4/1
  front unsprung weight/1 -> Divide5/1, unsprung WT lateral/4(front unsprung weight)
  Constant/1 -> Divide5/2
  Divide5/1 -> Add2/4, Divide3/1, Sum/1
  Constant4/1 -> Divide6/2
  Divide6/1 -> Divide/1, Add/4, Sum/2  "F_gravity"
  Divide4/1 -> Integrator2/1  "a"
  Integrator2/1 -> Subtract2/2, Subtract3/1, Integrator3/1  "v"
  Integrator3/1 -> Subtract1/2, Add3/2  "x"
  front spring MR/1 -> Product4/1, Product1/2
  front roll bar MR/1 -> Product2/3
  Product2/1 -> Add/3
  Product4/1 -> Add2/3, Add/5
  Product1/1 -> Add2/2, Add/2
  road height/1 -> Add3/1, elastic sprung WT lateral/6(road height)
  front tire stiffness/1 -> Product/2
  Product/1 -> Add2/6
  road velocity/1 -> Subtract3/2
  Subtract3/1 -> Product3/2
  front tire damping/1 -> Product3/1
  Constant5/1 -> Switch/3
  Switch/1 -> Product/1
  Add3/1 -> Gain/1, Switch/1, Switch/2, Switch1/2
  Constant6/1 -> Switch1/3
  Product3/1 -> Switch1/1
  Switch1/1 -> Add2/5
  Subtract1/1 -> Switch3/2, Switch2/1, Switch2/2
  Constant7/1 -> Switch2/3
  Switch2/1 -> Product1/3
  Constant8/1 -> Switch3/3
  Switch3/1 -> Product4/2
  Add/1 -> Divide2/1
  Sum/1 -> Fz_RR/1
  Sum1/1 -> Subtract/1, rear sprung mass offset/1, sprung height RR/1
  Subtract2/1 -> Switch3/1
  CG front/1 -> elastic sprung WT longitudinal/6(CG front)
  elastic sprung WT lateral/1(elastic lat WT) -> F1/2
  chassis force/1 -> Add/6
  Gain/1 -> Sum1/1

== system car_sim/Front/FL/ unsprung WT longitudinal ==
  longitudinal a : Inport
  wheelbase : Inport  Port=2
  front unsprung weight cg height : Inport  Port=3
  total unsprung weight : Inport  Port=4
  Constant : Constant  Value=32.17
  Divide : Product  Inputs=*/
  Divide1 : Product  Inputs=*/
  Product : Product  Inputs=3
  long WT : Outport
  wires:
  Divide/1 -> long WT/1
  Product/1 -> Divide/1
  longitudinal a/1 -> Product/1
  front unsprung weight cg height/1 -> Product/3
  total unsprung weight/1 -> Divide1/1
  Constant/1 -> Divide1/2
  Divide1/1 -> Product/2  "mass"
  wheelbase/1 -> Divide/2

== system car_sim/Front/FL/elastic sprung WT lateral ==
  CG h : Inport
  lateral a : Inport  Port=2
  track : Inport  Port=3
  front RC : Inport  Port=4
  front sprung weight : Inport  Port=5
  road height : Inport  Port=6
  Divide : Product  Inputs=*/
  Divide1 : Product  Inputs=*/
  Divide2 : Product  Inputs=*/
  Product : Product  Inputs=3
  Product1 : Product  Inputs=3
  Subtract : Sum  Inputs=+-
  Sum : Sum  Inputs=|++
  g : Constant  Value=32.17
  elastic lat WT : Outport
  geom lat WT : Outport  Port=2
  wires:
  Divide/1 -> elastic lat WT/1
  track/1 -> Divide2/2, Divide/2
  Product/1 -> Divide/1
  CG h/1 -> Subtract/1
  Subtract/1 -> Product/3
  lateral a/1 -> Product1/2, Product/1
  front sprung weight/1 -> Divide1/1
  g/1 -> Divide1/2
  Divide1/1 -> Product1/3, Product/2  "mass"
  Product1/1 -> Divide2/1
  Divide2/1 -> geom lat WT/1
  road height/1 -> Sum/1
  Sum/1 -> Subtract/2
  front RC/1 -> Sum/2, Product1/1

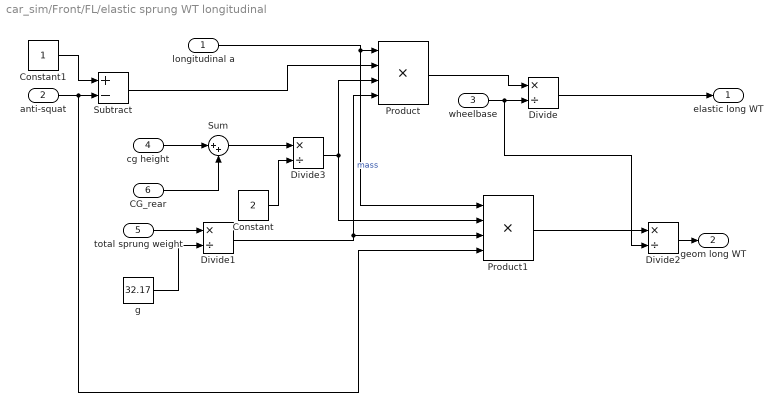
== system car_sim/Front/FL/elastic sprung WT longitudinal ==
  longitudinal a : Inport
  anti-squat : Inport  Port=2
  wheelbase : Inport  Port=3
  cg height : Inport  Port=4
  total sprung weight : Inport  Port=5
  CG_rear : Inport  Port=6
  Constant : Constant  Value=2
  Constant1 : Constant
  Divide{,1..3} (4 alike) : Product  Inputs=*/
  Product : Product  Inputs=4
  Product1 : Product  Inputs=4
  Subtract : Sum  Inputs=+-
  Sum : Sum  Inputs=|++
  g : Constant  Value=32.17
  elastic long WT : Outport
  geom long WT : Outport  Port=2
  wires:
  Product/1 -> Divide/1
  longitudinal a/1 -> Product1/1, Product/1
  anti-squat/1 -> Product1/4, Subtract/2
  Constant1/1 -> Subtract/1
  Subtract/1 -> Product/2
  total sprung weight/1 -> Divide1/1
  g/1 -> Divide1/2
  Divide1/1 -> Product/4, Product1/3  "mass"
  wheelbase/1 -> Divide2/2, Divide/2
  Divide2/1 -> geom long WT/1
  Product1/1 -> Divide2/1
  Divide/1 -> elastic long WT/1
  cg height/1 -> Sum/1
  CG_rear/1 -> Sum/2
  Sum/1 -> Divide3/1
  Constant/1 -> Divide3/2
  Divide3/1 -> Product/3, Product1/2

== system car_sim/Front/FL/unsprung WT lateral ==
  front unsprung cg height : Inport
  lateral a : Inport  Port=2
  track : Inport  Port=3
  front unsprung weight : Inport  Port=4
  Divide : Product  Inputs=*/
  Divide1 : Product  Inputs=*/
  Product : Product  Inputs=3
  g : Constant  Value=32.17
  lat WT : Outport
  wires:
  Divide/1 -> lat WT/1
  Product/1 -> Divide/1
  lateral a/1 -> Product/1
  front unsprung weight/1 -> Divide1/1
  g/1 -> Divide1/2
  Divide1/1 -> Product/2
  front unsprung cg height/1 -> Product/3
  track/1 -> Divide/2

== system car_sim/Front/FR/ unsprung WT longitudinal ==
  longitudinal a : Inport
  wheelbase : Inport  Port=2
  front unsprung weight cg height : Inport  Port=3
  total unsprung weight : Inport  Port=4
  Constant : Constant  Value=32.17
  Divide : Product  Inputs=*/
  Divide1 : Product  Inputs=*/
  Product : Product  Inputs=3
  long WT : Outport
  wires:
  Divide/1 -> long WT/1
  Product/1 -> Divide/1
  longitudinal a/1 -> Product/1
  front unsprung weight cg height/1 -> Product/3
  total unsprung weight/1 -> Divide1/1
  Constant/1 -> Divide1/2
  Divide1/1 -> Product/2  "mass"
  wheelbase/1 -> Divide/2

== system car_sim/Front/FR/elastic sprung WT lateral ==
  CG h : Inport
  lateral a : Inport  Port=2
  track : Inport  Port=3
  front RC : Inport  Port=4
  front sprung weight : Inport  Port=5
  road height : Inport  Port=6
  Divide : Product  Inputs=*/
  Divide1 : Product  Inputs=*/
  Divide2 : Product  Inputs=*/
  Product : Product  Inputs=3
  Product1 : Product  Inputs=3
  Subtract : Sum  Inputs=+-
  Sum : Sum  Inputs=|++
  g : Constant  Value=32.17
  elastic lat WT : Outport
  geom lat WT : Outport  Port=2
  wires:
  Divide/1 -> elastic lat WT/1
  track/1 -> Divide2/2, Divide/2
  Product/1 -> Divide/1
  CG h/1 -> Subtract/1
  Subtract/1 -> Product/3
  lateral a/1 -> Product1/2, Product/1
  front sprung weight/1 -> Divide1/1
  g/1 -> Divide1/2
  Divide1/1 -> Product1/3, Product/2  "mass"
  Product1/1 -> Divide2/1
  Divide2/1 -> geom lat WT/1
  front RC/1 -> Product1/1, Sum/2
  road height/1 -> Sum/1
  Sum/1 -> Subtract/2
